simulink model "simulink_model_closedloop"  (R2021b)
settings: Solver=FixedStepAuto  StartTime=0.0  StopTime=Tf  FixedStep=0.02  RelTol=1e-3
values from neighbouring files (symbols this model uses):
  constraint = struct()    [bicycle_model.m]
  model = struct()    [bicycle_model.m]
  N = 50    [main_for_simulink.m]    (also in main_for_simulink_delete.m)
settings Model: Creator=oj  LastModifiedBy=Hongbin
settings SolverCC: AlgebraicLoopSolver=TrustRegion
settings DataIOCC: SaveFormat=StructureWithTime  ReturnWorkspaceOutputs=off
settings OptimizationCC: LifeSpan=inf
settings DebuggingCC: SFExecutionAtInitializationDiag=none  SFMachineParentedDataDiag=warning  ArithmeticOperatorsInVariantConditions=warning
settings HardwareCC: ProdBitPerSizeT=32  ProdBitPerPtrDiffT=32  ProdWordSize=32  ProdHWDeviceType=Specified
settings SFSimCC: CustomCodeUndefinedFunction=UseInterfaceOnly
settings CodeAppCC: StateflowObjectComments=on

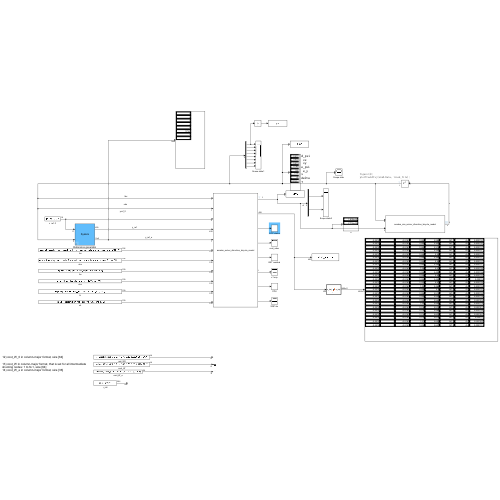
[thumbnail: Simulink's stored preview of the top-level diagram]
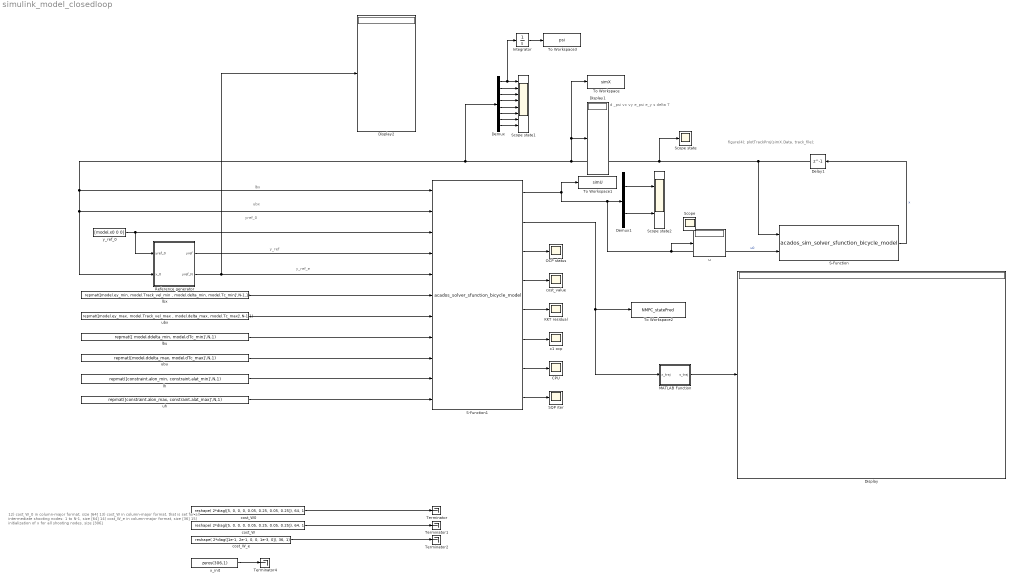
== system simulink_model_closedloop ==
  note: 12) cost_W_0 in column-major format, size [64]
      |
      | 13) cost_W in column-major format, that is set for all intermediate shooting nodes: 1 to N-1, size [64]
      | 14) cost_W_e in column-major format, size [36]
      | 15) initialization of x for all shooting nodes, size [306]
  note: yref_0
  note: ubx
  note: lbx
  note: figure(4);
      | plotTrackProj(simX.Data, track_file);
  note: y_ref_e
  note: y_ref
  note: d _psi
      | vx
      | vy
      | e_psi
      | e_y
      | s
      | delta
      | T
  CPU : Scope
      settings: Description=status
  Delay1 : Delay  DelayLength=1  InitialCondition=model.x0
  Demux : Demux  Outputs=8
  Demux1 : Demux  Outputs=2
  Display : Display
  Display1 : Display
  Display2 : Display
  Integrator : Integrator
  KKT residual : Scope
      settings: Description=status
  MATLAB Function : MATLAB Function  TreatAsAtomicUnit=on
  OCP status : Scope
      settings: Description=status
  Reference generator : Subsystem
      mask help: Simple system simulation.
      mask init:
      | % initialize state values
      mask Display: disp('System');
  S-Function : S-Function  FunctionName=acados_sim_solver_sfunction_bicycle_model  SFunctionDeploymentMode=off  EnableBusSupport=off
  S-Function1 : S-Function  FunctionName=acados_solver_sfunction_bicycle_model  SFunctionDeploymentMode=off  EnableBusSupport=off
  SQP iter : Scope
      settings: Description=status
  Scope state : Scope
  Scope state1 : Scope  NumInputPorts=8
  Scope state2 : Scope  NumInputPorts=2
  Terminator{,1..2,4} (4 alike) : Terminator
  To Workspace : ToWorkspace  VariableName=simX  SaveFormat=Timeseries  SampleTime=-1
  To Workspace1 : ToWorkspace  VariableName=simU  SaveFormat=Timeseries  SampleTime=-1
  To Workspace2 : ToWorkspace  VariableName=NMPC_statePred  SaveFormat=Structure  SampleTime=-1
  To Workspace3 : ToWorkspace  VariableName=psi  SaveFormat=Timeseries  SampleTime=-1
  cost_W : Constant  Value=reshape( 2*diag([5, 0, 0, 0, 0.05, 0.25, 0.05, 0.25]), 64, 1)
  cost_W0 : Constant  Value=reshape( 2*diag([5, 0, 0, 0, 0.05, 0.25, 0.05, 0.25]), 64, 1)
  cost_W_e : Constant  Value=reshape( 2*diag([1e-1, 2e-1, 0, 0, 1e-3, 0]), 36, 1)
  cost_value : Scope
      settings: Description=status
  lbu : Constant  Value=repmat([ model.ddelta_min, model.dTc_min]',N,1)
  lbx : Constant  Value=repmat([model.ey_min, model.Track_vel_min , model.delta_min, model.Tc_min]',N-1,1)
  lh : Constant  Value=repmat([constraint.alon_min, constraint.alat_min]',N,1)
  u : Display
  ubu : Constant  Value=repmat([model.ddelta_max, model.dTc_max]',N,1)
  ubx : Constant  Value=repmat([model.ey_max, model.Track_vel_max , model.delta_max, model.Tc_max]',N-1,1)
  uh : Constant  Value=repmat([constraint.alon_max, constraint.alat_max]',N,1)
  x1 ocp : Scope
      settings: Description=status
  x_init : Constant  Value=zeros(306,1)
  y_ref_0 : Constant  Value=[model.x0 0 0]
  Scope : Scope
  wires:
  S-Function/1 -> Delay1/1  "x"
  lbu/1 -> S-Function1/8
  lh/1 -> S-Function1/10
  uh/1 -> S-Function1/11
  Demux/6 -> Scope state1/6
  Demux/5 -> Scope state1/5
  Demux/4 -> Scope state1/4
  Demux/3 -> Scope state1/3
  Demux/1 -> Integrator/1, Scope state1/1
  S-Function1/1 -> Demux1/1, u/1, S-Function/2, To Workspace1/1  "u0"
  Delay1/1 -> S-Function/1, Demux/1, Reference generator/2(x_0), S-Function1/2, S-Function1/1, To Workspace/1, Display1/1, Scope state/1
  y_ref_0/1 -> S-Function1/3, Reference generator/1(yref_0)
  Reference generator/1(yref) -> S-Function1/4
  Demux1/1 -> Scope state2/1
  Demux1/2 -> Scope state2/2
  Demux/2 -> Scope state1/2
  ubx/1 -> S-Function1/7
  cost_W/1 -> Terminator1/1
  cost_W0/1 -> Terminator/1
  cost_W_e/1 -> Terminator2/1
  x_init/1 -> Terminator4/1
  Demux/7 -> Scope state1/7
  Demux/8 -> Scope state1/8
  MATLAB Function/1(s_traj) -> Display/1
  S-Function1/2 -> To Workspace2/1, MATLAB Function/1(x_traj)
  Reference generator/2(yref_N) -> Display2/1, S-Function1/5
  lbx/1 -> S-Function1/6
  ubu/1 -> S-Function1/9
  S-Function1/5 -> KKT residual/1
  S-Function1/6 -> x1 ocp/1
  S-Function1/7 -> CPU/1
  S-Function1/8 -> SQP iter/1
  S-Function1/3 -> OCP status/1
  S-Function1/4 -> cost_value/1
  Integrator/1 -> To Workspace3/1

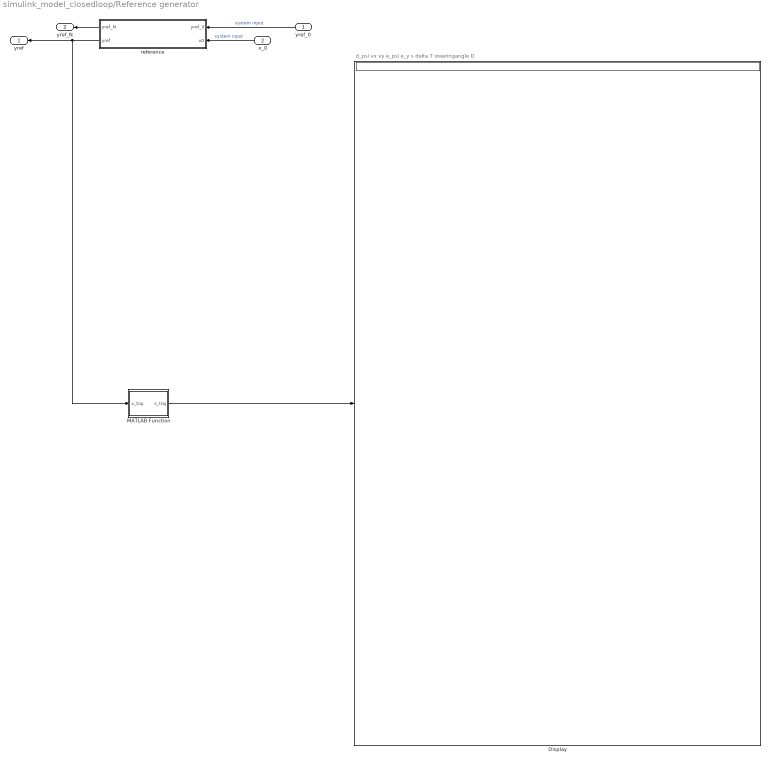
== system simulink_model_closedloop/Reference generator ==
  note: d_psi vx vy e_psi e_y s delta T steeringangle D
  yref_0 : Inport
  x_0 : Inport  Port=2
  Display : Display
  MATLAB Function : MATLAB Function  TreatAsAtomicUnit=on
  reference : MATLAB Function  TreatAsAtomicUnit=on
  yref : Outport
  yref_N : Outport  Port=2
  wires:
  reference/2(yref) -> MATLAB Function/1(x_traj), yref/1
  reference/1(yref_N) -> yref_N/1
  x_0/1 -> reference/2(x0)  "system input"
  yref_0/1 -> reference/1(yref_0)  "system input"
  MATLAB Function/1(s_traj) -> Display/1

== matlab function simulink_model_closedloop/MATLAB Function ==
  data: x_traj input; s_traj output
function s_traj = fcn(x_traj)

nx = 9;
s_traj = x_traj(9:408);

== matlab function simulink_model_closedloop/Reference generator/reference ==
  data: yref_0 input; x0 input; yref_N output; yref output
function [yref_N, yref] = Generate_reference(yref_0, x0)
s0 = x0(6);
sref_N = 3;  % reference for final reference progress
N = 50;
sref = s0 + sref_N;

% yref =repmat(zeros(size(yref_0,1),1),N-1,1);
yref =repmat([0 0 0 0 0 0 0 0 0 0]',N-1,1);
    for j = 1:(N-1)
        yref(6+(j-1)*size(yref_0,1)) = s0 + (sref - s0) * j / N;
            
    end

yref_N = [0, 0, 0, 0, 0, sref,0,0];

== matlab function simulink_model_closedloop/Reference generator/MATLAB Function ==
  data: x_traj input; s_traj output
function s_traj = fcn(x_traj)

nx = 7/7;
% s_traj =zeros(51,1);
s_traj = x_traj(1:nx:490);
